simulink model "L5A2"  (R2021b)
settings: Solver=VariableStepAuto  StartTime=0.0  StopTime=10.0  RelTol=1e-3
undefined symbols (not defined in the file): c_i, c_y, K_r, L, m, R
settings Model: Creator=tobia  LastModifiedBy=tobia

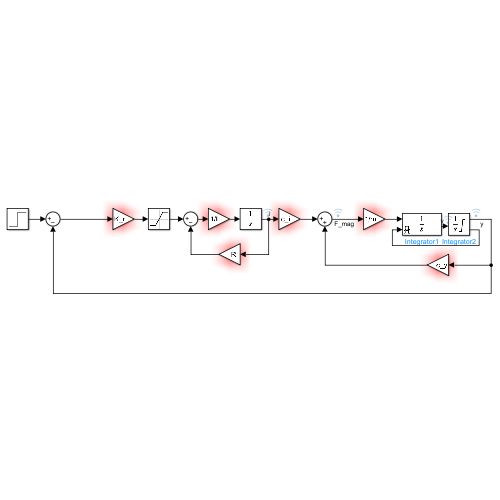
[thumbnail: Simulink's stored preview of the top-level diagram]
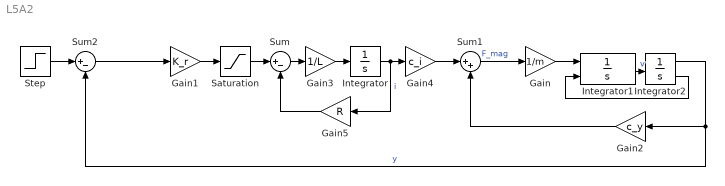
== system L5A2 ==
  Gain : Gain  Gain=1/m
  Gain1 : Gain  Gain=K_r
  Gain2 : Gain  Gain=c_y
  Gain3 : Gain  Gain=1/L
  Gain4 : Gain  Gain=c_i
  Gain5 : Gain  Gain=R
  Integrator : Integrator
  Integrator1 : Integrator  ExternalReset=either
  Integrator2 : Integrator  InitialCondition=-1e-3  LimitOutput=on  UpperSaturationLimit=5e-3  LowerSaturationLimit=-5e-2  ShowSaturationPort=on
  Saturation : Saturate  UpperLimit=6  LowerLimit=-6
  Step : Step  Time=0  After=0  SampleTime=0
  Sum : Sum  Inputs=|+-
  Sum1 : Sum  Inputs=|++
  Sum2 : Sum  Inputs=|+-
  wires:
  Gain/1 -> Integrator1/1
  Integrator1/1 -> Integrator2/1  "v"
  Sum/1 -> Gain3/1
  Gain3/1 -> Integrator/1
  Integrator/1 -> Gain4/1, Gain5/1  "i"
  Gain4/1 -> Sum1/1
  Sum1/1 -> Gain/1  "F_mag"
  Integrator2/1 -> Gain2/1, Sum2/2  "y"
  Gain2/1 -> Sum1/2
  Gain5/1 -> Sum/2
  Step/1 -> Sum2/1
  Sum2/1 -> Gain1/1
  Gain1/1 -> Saturation/1
  Saturation/1 -> Sum/1
  Integrator2/2 -> Integrator1/2
